simulink library "INT_AirCtl_Co"  (R2016b)
settings: Solver=VariableStepAuto  StartTime=0.0  StopTime=10.0  RelTol=1e-3
settings Model: Creator=zhulinfeng  LastModifiedBy=zhulinfeng

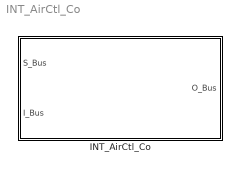
== system INT_AirCtl_Co ==
  INT_AirCtl_Co : Subsystem

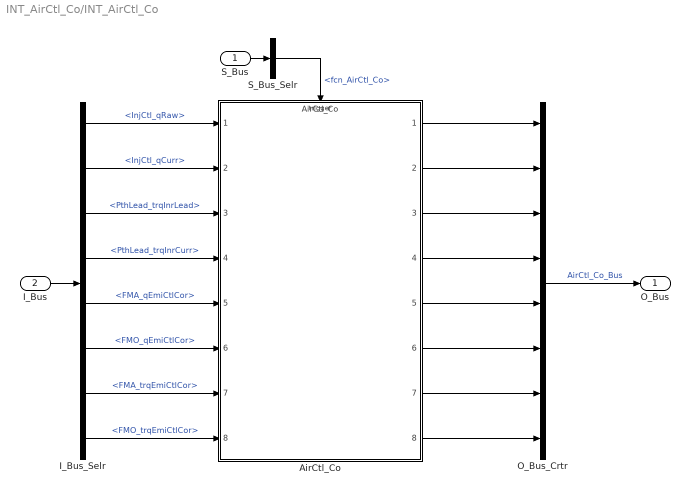
== system INT_AirCtl_Co/INT_AirCtl_Co ==
  S_Bus : Inport
  I_Bus : Inport  Port=2
  AirCtl_Co : ModelReference  ModelNameDialog=AirCtl_Co  SimulationMode=Normal  ModelReferenceVersion=1.15  TriggerPortName=function  TriggerPortTriggerType=function-call  TriggerPortStatesWhenEnabling=held
  I_Bus_Selr : BusSelector  OutputSignals=InjCtl_qRaw,InjCtl_qCurr,PthLead_trqInrLead,PthLead_trqInrCurr,FMA_qEmiCtlCor,FMO_qEmiCtlCor,FMA_trqEmiCtlCor,FMO_trqEmiCtlCor
  O_Bus_Crtr : BusCreator  Inputs=8
  S_Bus_Selr : BusSelector  OutputSignals=fcn_AirCtl_Co
  O_Bus : Outport
  wires:
  S_Bus_Selr/1 -> AirCtl_Co/Trigger  "<fcn_AirCtl_Co>"
  S_Bus/1 -> S_Bus_Selr/1
  I_Bus/1 -> I_Bus_Selr/1
  I_Bus_Selr/1 -> AirCtl_Co/1  "<InjCtl_qRaw>"
  I_Bus_Selr/2 -> AirCtl_Co/2  "<InjCtl_qCurr>"
  I_Bus_Selr/3 -> AirCtl_Co/3  "<PthLead_trqInrLead>"
  I_Bus_Selr/4 -> AirCtl_Co/4  "<PthLead_trqInrCurr>"
  I_Bus_Selr/5 -> AirCtl_Co/5  "<FMA_qEmiCtlCor>"
  I_Bus_Selr/6 -> AirCtl_Co/6  "<FMO_qEmiCtlCor>"
  I_Bus_Selr/7 -> AirCtl_Co/7  "<FMA_trqEmiCtlCor>"
  I_Bus_Selr/8 -> AirCtl_Co/8  "<FMO_trqEmiCtlCor>"
  O_Bus_Crtr/1 -> O_Bus/1  "AirCtl_Co_Bus"
  AirCtl_Co/1 -> O_Bus_Crtr/1
  AirCtl_Co/2 -> O_Bus_Crtr/2
  AirCtl_Co/3 -> O_Bus_Crtr/3
  AirCtl_Co/4 -> O_Bus_Crtr/4
  AirCtl_Co/5 -> O_Bus_Crtr/5
  AirCtl_Co/6 -> O_Bus_Crtr/6
  AirCtl_Co/7 -> O_Bus_Crtr/7
  AirCtl_Co/8 -> O_Bus_Crtr/8
